simulink model "Sim_model_2019a"  (R2019a)
settings: Solver=FixedStepAuto  StartTime=0.0  StopTime=350  FixedStep=0.5  RelTol=1e-3
libraries: mpclib x1
settings Model: Creator=USER  LastModifiedBy=USER

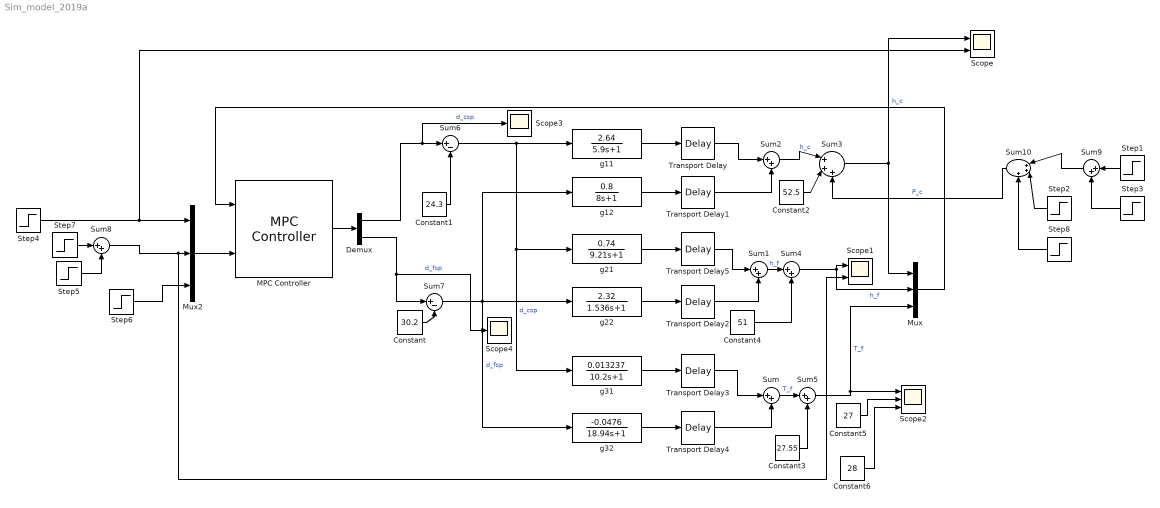
== system Sim_model_2019a ==
  Constant : Constant  Value=30.2
  Constant1 : Constant  Value=24.3
  Constant2 : Constant  Value=52.5
  Constant3 : Constant  Value=27.55
  Constant4 : Constant  Value=51
  Constant5 : Constant  Value=27
  Constant6 : Constant  Value=28
  Demux : Demux  Outputs=2
  MPC Controller : mpclib/MPC Controller  SCDEnableBlockLinearizationSpecification=on  mpcobj=mpcobj  is_multiple=0  enable_value=0  return_u0=off  updateMPCinCallerWorkspace=on  md_inport=off  mv_inport=off  uref_inport=off  return_cost=off  return_mvseq=off  return_qpstatus=off  return_xseq=off  return_state=off  return_ovseq=off  state_inport=off  umin_inport=off  umax_inport=off  ymin_inport=off  ymax_inport=off  cc_inport=off  ywt_inport=off  uwt_inport=off  duwt_inport=off  rhoeps_inport=off  pm_inport=off  MaximumP=20  HorizonChoice=FixedHorizon  n_ts=0.5  n_p=20  n_mv=2  n_md=0  n_ud=0  n_mo=3  n_uo=0  BlockDataType=double  SampleTimeInherited=off  switch_inport=off
  Mux : Mux  Inputs=3
  Mux2 : Mux  Inputs=3
  Scope : Scope  NumInputPorts=2
  Scope1 : Scope  NumInputPorts=2
  Scope2 : Scope  NumInputPorts=3
  Scope3 : Scope
  Scope4 : Scope
  Step1 : Step  Time=300  After=25  SampleTime=0
  Step2 : Step  Time=50  After=-25  SampleTime=0
  Step3 : Step  Time=200  After=-25  SampleTime=0
  Step4 : Step  Time=150  Before=52.5  After=52.5+25  SampleTime=0
  Step5 : Step  Time=5  Before=51  After=51+10  SampleTime=0
  Step6 : Step  Time=0  After=0  SampleTime=0
  Step7 : Step  Time=150  After=-10  SampleTime=0
  Step8 : Step  Time=100  After=25  SampleTime=0
  Sum{,1..2,4..5,8..9} (7 alike) : Sum  Inputs=|++
  Sum10 : Sum  Inputs=|+++
  Sum3 : Sum  Inputs=|+++
  Sum6 : Sum  Inputs=|+-
  Sum7 : Sum  Inputs=|+-
  Transport Delay : TransportDelay  DelayTime=2.5
  Transport Delay1 : TransportDelay
  Transport Delay2 : TransportDelay  DelayTime=3
  Transport Delay3 : TransportDelay  DelayTime=2
  Transport Delay4 : TransportDelay  DelayTime=3.5
  Transport Delay5 : TransportDelay  DelayTime=.5
  g11 : TransferFcn  Numerator=2.64  Denominator=[5.9 1]
  g12 : TransferFcn  Numerator=0.8  Denominator=[8 1]
  g21 : TransferFcn  Numerator=0.74  Denominator=[9.21 1]
  g22 : TransferFcn  Numerator=2.32  Denominator=[1.536 1]
  g31 : TransferFcn  Numerator=[0.013237]  Denominator=[10.2 1]
  g32 : TransferFcn  Numerator=[-0.0476]  Denominator=[18.94 1]
  wires:
  g11/1 -> Transport Delay/1
  g12/1 -> Transport Delay1/1
  g22/1 -> Transport Delay2/1
  g31/1 -> Transport Delay3/1
  Transport Delay3/1 -> Sum/1
  Transport Delay4/1 -> Sum/2
  Sum/1 -> Sum5/1  "T_f"
  Transport Delay2/1 -> Sum1/2
  Transport Delay/1 -> Sum2/1
  Transport Delay1/1 -> Sum2/2
  MPC Controller/1 -> Demux/1
  Mux/1 -> MPC Controller/1
  g32/1 -> Transport Delay4/1
  Sum5/1 -> Mux/3, Scope2/1  "T_f"
  Demux/1 -> Scope3/1, Sum6/1  "d_csp"
  Constant1/1 -> Sum6/2
  Sum6/1 -> g11/1, g21/1, g31/1  "d_csp"
  Demux/2 -> Sum7/1, Scope4/1  "d_fsp"
  Constant/1 -> Sum7/2
  Sum7/1 -> g12/1, g32/1, g22/1  "d_fsp"
  Sum2/1 -> Sum3/1  "h_c"
  Constant2/1 -> Sum3/2
  Sum3/1 -> Scope/1, Mux/1  "h_c"
  Sum1/1 -> Sum4/1  "h_f"
  Sum4/1 -> Mux/2, Scope1/1  "h_f"
  Constant4/1 -> Sum4/2
  Constant3/1 -> Sum5/2
  Step4/1 -> Scope/2, Mux2/1
  Step5/1 -> Sum8/2
  Mux2/1 -> MPC Controller/2
  Sum8/1 -> Scope1/2, Mux2/2
  Step6/1 -> Mux2/3
  Step7/1 -> Sum8/1
  Constant5/1 -> Scope2/2
  Constant6/1 -> Scope2/3
  Step1/1 -> Sum9/1
  Step3/1 -> Sum9/2
  Sum9/1 -> Sum10/1
  Step2/1 -> Sum10/2
  Step8/1 -> Sum10/3
  Sum10/1 -> Sum3/3  "P_c"
  g21/1 -> Transport Delay5/1
  Transport Delay5/1 -> Sum1/1
